simulink model "AutomotiveEMS"  (R2018a)
settings: Solver=VariableStepAuto  StartTime=0  StopTime=3.5  FixedStep=1e-6
undefined symbols (not defined in the file): alternator, buck, DiscIntNeverNeededParam, electrical_load, hybrid_control, i_f_max, iceToAltRotRatio, n_ice_f, n_ice_i, rectifier, t_brake_f, t_brake_i, T_k, T_r, T_s
libraries: fl_lib x43, nesl_utility x41, elec_lib x33, simulink x10, SimscapeCustomBlocks_lib x2, dsparch4 x2, pe_lib x1
(part 1 of 3)
settings Model: Creator=gabrielrodrigues  LastModifiedBy=gabriel.rodrigues
settings DataIOCC: ReturnWorkspaceOutputs=on
settings CodeAppCC: StateflowObjectComments=on
settings SimscapeCC: SimscapeNormalizeSystem=off  SimscapeLogType=local  SimscapeLogLimitData=off

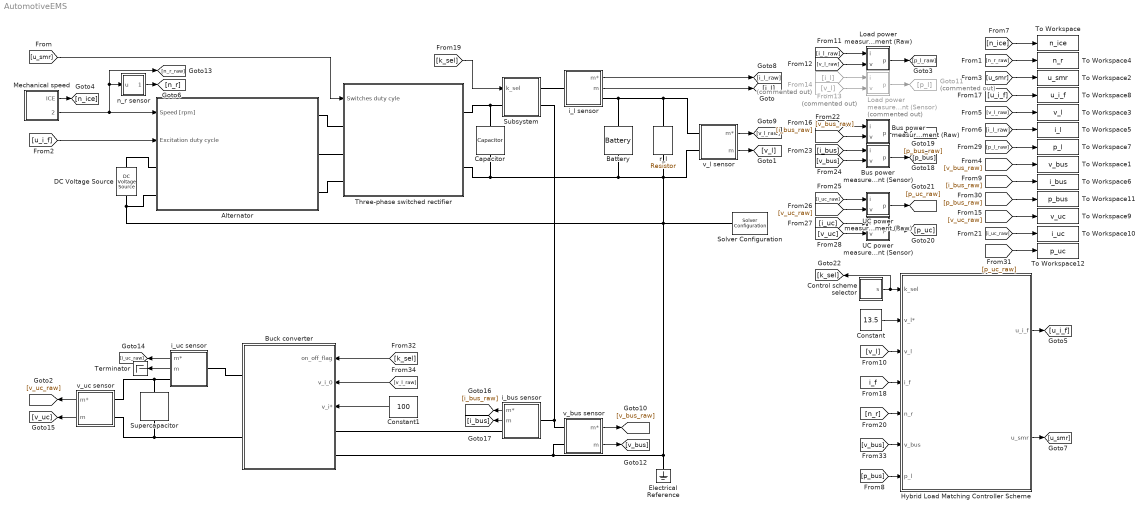
== system AutomotiveEMS ==
  Alternator : Subsystem
  Battery : elec_lib/Sources/Battery  Vnom=battery.v_nom V  R1=battery.r Ohm  prm_AH=2  AH=120 hr*A  V1=11.5 V  AH1=25 hr*A  prm_R2=1  R2=2000 Ohm  prm_dyn=1  Rp1=0.005 Ohm  tau1=30 s  Rp2=0.005 Ohm  tau2=30 s  Rp3=0.005 Ohm  tau3=30 s  Rp4=0.005 Ohm  tau4=30 s  Rp5=0.005 Ohm  tau5=30 s  prm_fade=1  N_fade=100  AH_fade=45 hr*A  R1_fade=2.02 Ohm  V1_fade=10.35 V  i_specify=off  i_priority=None  i=0 A  i_nominal_specify=off  i_nominal_unit=A  i_nominal_value=1  v_specify=off  v_priority=None  v=0 V  v_nominal_specify=off  v_nominal_unit=V  v_nominal_value=1  charge_specify=off  charge_priority=High  charge=50 hr*A  charge_nominal_specify=off  charge_nominal_unit=hr*A  charge_nominal_value=1  num_cycles_specify=off  num_cycles_priority=High  num_cycles=0  num_cycles_nominal_specify=off  num_cycles_nominal_unit=1  num_cycles_nominal_value=1  thermal_mass=30000 J/K  Tmeas=298.15 K  Vnom_T2=12 V  R1_T2=2.2 Ohm  V1_T2=11.4 V  R2_T2=2200 Ohm  Rp1_T2=0.005 Ohm  tau1_T2=30 s  Rp2_T2=0.005 Ohm  tau2_T2=30 s  Rp3_T2=0.005 Ohm  tau3_T2=30 s  Rp4_T2=0.005 Ohm  tau4_T2=30 s  Rp5_T2=0.005 Ohm  tau5_T2=30 s  Tmeas2=273.15 K  temperature_specify=off  temperature_priority=High  temperature=298.15 K  temperature_nominal_specify=off  temperature_nominal_unit=K  temperature_nominal_value=1
      settings: SourceProductName=Simscape Electronics  SourceProductBaseCode=SN
  Buck converter : Subsystem  mask{eta=buck.efficiency, v_o_max=buck.v_o_max}
      mask prompts: eta "Converter efficiency"; v_o_max "Maximum output voltage [V]"
  Bus power measurement (Raw) : Subsystem
  Bus power measurement (Sensor) : Subsystem
  Capacitor : fl_lib/Electrical/Electrical Elements/Capacitor  c=rectifier.filter.c F  r=1e-6 Ohm  g=0 1/Ohm  i_specify=off  i_priority=None  i=0 A  i_nominal_specify=off  i_nominal_unit=A  i_nominal_value=1  v_specify=off  v_priority=None  v=0 V  v_nominal_specify=off  v_nominal_unit=V  v_nominal_value=1  vc_specify=off  vc_priority=High  vc=0 V  vc_nominal_specify=off  vc_nominal_unit=V  vc_nominal_value=1
  Constant : Constant  Value=13.5
  Constant1 : Constant  Value=100
  Control scheme selector : Subsystem  mask{s_i=0, s_f=1, t_i=t_brake_i, t_f=t_brake_f}
      mask prompts: s_i "Initial value"; s_f "Final value"; t_i "Step start [s]"; t_f "Step end [s]"
  DC Voltage Source : elec_lib/Additional Components/SPICE-Compatible Components/Sources/DC Voltage Source  DC=alternator.rotor.r.value * i_f_max V
      settings: SourceProductName=Simscape Electronics  SourceProductBaseCode=SN
  Electrical Reference : fl_lib/Electrical/Electrical Elements/Electrical Reference
  From13 : From  Commented=on  GotoTag=i_l
  From14 : From  Commented=on  GotoTag=v_l
  Goto11 : Goto  Commented=on  GotoTag=p_l
  Hybrid Load Matching Controller Scheme : Subsystem  VariantControl=neural3InControlScheme
  Load power measurement (Raw) : Subsystem
  Load power measurement (Sensor) : Subsystem  Commented=on
  Mechanical speed : Subsystem
  Solver Configuration : nesl_utility/Solver Configuration  PhysicalDomain=network_engine_domain  SubClassName=solver  LeftPortType=input  RightPortType=generic  Tones=[]  Harmonics=[]  SimulateNoise=off  Profile=off  UseLocalSampling=off  EnableSwitchedLinearOptims=on  FrequencyDomain=off  UseCCode=off  RelTol=0.001  AbsTol=1e-06  MinStep=1e-09  ToWorkspace=off  RevertToSquareIcSolve=off  NumHomotopyIterations=100  PhasorMode=off  PhasorModeNumHarmonics=1  DoDC=off  ResidualTolerance=1e-09  UseLocalSolver=on  LocalSolverChoice=NE_TRAPEZOIDAL_ADVANCER  LocalSolverSampleTime=1e-06  DoFixedCost=on  MaxNonlinIter=20  MaxModeIter=2  LinearAlgebra=Sparse  EquationFormulation=NE_TIME_EF  DelaysMemoryBudget=1024  AutomaticFiltering=on  FilteringTimeConstant=0.001  PartitionStorageMethod=AS_NEEDED  PartitionMemoryBudget=1024
  Subsystem : Subsystem
  Supercapacitor : pe_lib/Sources/Supercapacitor  R=[1.5e-3, 0.4, 3.2] Ohm  C=[900, 200, 330] F  Kv=600 F/V  R_discharge=4e+3 Ohm  N_series=6  N_parallel=4  i_specify=off  i_priority=None  i=0 A  i_nominal_specify=off  i_nominal_unit=A  i_nominal_value=1  v_specify=off  v_priority=None  v=0 V  v_nominal_specify=off  v_nominal_unit=V  v_nominal_value=1  vc1_specify=off  vc1_priority=High  vc1=0 V  vc1_nominal_specify=off  vc1_nominal_unit=V  vc1_nominal_value=1  vc2_specify=off  vc2_priority=High  vc2=0 V  vc2_nominal_specify=off  vc2_nominal_unit=V  vc2_nominal_value=1  vc3_specify=off  vc3_priority=High  vc3=0 V  vc3_nominal_specify=off  vc3_nominal_unit=V  vc3_nominal_value=1
      settings: SourceProductName=Simscape Electrical  SourceProductBaseCode=PS
  Terminator : Terminator
  Three-phase switched rectifier : Subsystem
  To Workspace : ToWorkspace  VariableName=n_ice  SaveFormat=Timeseries  SampleTime=-1
  To Workspace1 : ToWorkspace  VariableName=v_bus  SaveFormat=Timeseries  SampleTime=-1
  To Workspace10 : ToWorkspace  VariableName=i_uc  SaveFormat=Timeseries  SampleTime=-1
  To Workspace11 : ToWorkspace  VariableName=p_bus  SaveFormat=Timeseries  SampleTime=-1
  To Workspace12 : ToWorkspace  VariableName=p_uc  SaveFormat=Timeseries  SampleTime=-1
  To Workspace2 : ToWorkspace  VariableName=u_smr  SaveFormat=Timeseries  SampleTime=-1
  To Workspace3 : ToWorkspace  VariableName=v_l  SaveFormat=Timeseries  SampleTime=-1
  To Workspace4 : ToWorkspace  VariableName=n_r  SaveFormat=Timeseries  SampleTime=-1
  To Workspace5 : ToWorkspace  VariableName=i_l  SaveFormat=Timeseries  SampleTime=-1
  To Workspace6 : ToWorkspace  VariableName=i_bus  SaveFormat=Timeseries  SampleTime=-1
  To Workspace7 : ToWorkspace  VariableName=p_l  SaveFormat=Timeseries  SampleTime=-1
  To Workspace8 : ToWorkspace  VariableName=u_i_f  SaveFormat=Timeseries  SampleTime=-1
  To Workspace9 : ToWorkspace  VariableName=v_uc  SaveFormat=Timeseries  SampleTime=-1
  UC power measurement (Raw) : Subsystem
  UC power measurement (Sensor) : Subsystem
  i_bus sensor : Subsystem
  i_l sensor : Subsystem
  i_uc sensor : Subsystem
  n_r sensor : Subsystem  mask{T_s=T_s, seed=1515, noise=0.001}
      mask prompts: T_s "Sample time [s]"; noise "Noise percentage"
      mask DialogControl DescGroupVar Prompt: Noisy voltage sensor
  r_l : elec_lib/Passive Devices/Resistor  R=electrical_load.r Ohm  R_tol=5  enable_R_tol=0  tol_distribution=1  nSigma=4  enable_operating_limits=0  operating_limit_action=2  max_working_voltage=100 V  power_rating=1 W  enable_faults=0  fault_action=1  R_faulted=inf Ohm  enable_temporal_fault=0  t_fault=1 s  enable_behavioral_fault=0  max_permissible_current=1 A  t_fail_on_current=1 s  noise_mode=0  sample_time=1e-3 s  repeatability=1  auto_seed=2238261350  user_seed=0  Tdevice=25 degC  alpha=3.93e-3 1/K  Tmeas=25 degC  thermal_mass=100 J/K  power_derating_T1=70 degC  power_derating_T2=155 degC  operating_temperature_range_vec=[-50, 150] degC  temperature_specify=off  temperature_priority=High  temperature=298.15 K  temperature_nominal_specify=off  temperature_nominal_unit=K  temperature_nominal_value=1
  v_bus sensor : Subsystem
  v_l sensor : Subsystem
  v_uc sensor : Subsystem
  wires:
  Mechanical speed/2(Alternator) -> Alternator/1(Speed [rpm]), [n_r_raw], n_r sensor/1(u)
  n_r sensor/1(m) -> [n_r]
  i_l sensor/2(m) -> [i_l]
  Hybrid Load Matching Controller Scheme/1(u_i_f) -> [u_i_f]
  v_l sensor/1(m*) -> [v_l_raw]
  [u_smr] -> Three-phase switched rectifier/1(Switches duty cyle)
  v_l sensor/2(m) -> [v_l]
  Hybrid Load Matching Controller Scheme/2(u_smr) -> [u_smr]
  Mechanical speed/1(ICE) -> [n_ice]
  i_l sensor/1(m*) -> [i_l_raw]
  [u_i_f] -> To Workspace8/1
  [u_smr] -> To Workspace2/1
  [v_l_raw] -> To Workspace3/1
  [n_ice] -> To Workspace/1
  [n_r_raw] -> To Workspace4/1
  [i_l_raw] -> To Workspace5/1
  [k_sel] -> Subsystem/1(k_sel)
  [p_bus] -> Hybrid Load Matching Controller Scheme/7(p_l)
  Constant/1 -> Hybrid Load Matching Controller Scheme/2(v_l*)
  [v_l] -> Hybrid Load Matching Controller Scheme/3(v_l)
  [n_r] -> Hybrid Load Matching Controller Scheme/5(n_r)
  Load power measurement (Sensor)/1(p) -> Goto11/1
  From13/1 -> Load power measurement (Sensor)/1(i)
  [v_l_raw] -> Load power measurement (Raw)/2(v)
  Load power measurement (Raw)/1(p) -> [p_l_raw]
  From14/1 -> Load power measurement (Sensor)/2(v)
  [i_l_raw] -> Load power measurement (Raw)/1(i)
  v_uc sensor/1(m*) -> [v_uc_raw]
  v_uc sensor/2(m) -> [v_uc]
  v_bus sensor/1(m*) -> [v_bus_raw]
  v_bus sensor/2(m) -> [v_bus]
  i_uc sensor/1(m*) -> [i_uc_raw]
  i_uc sensor/2(m) -> Terminator/1
  [i_bus_raw] -> To Workspace6/1
  [v_bus_raw] -> To Workspace1/1
  [i_uc_raw] -> To Workspace10/1
  [v_uc_raw] -> To Workspace9/1
  i_bus sensor/1(m*) -> [i_bus_raw]
  i_bus sensor/2(m) -> [i_bus]
  [i_bus_raw] -> Bus power measurement (Raw)/1(i)
  Bus power measurement (Raw)/1(p) -> [p_bus_raw]
  [v_bus] -> Bus power measurement (Sensor)/2(v)
  [v_bus_raw] -> Bus power measurement (Raw)/2(v)
  [i_bus] -> Bus power measurement (Sensor)/1(i)
  Bus power measurement (Sensor)/1(p) -> [p_bus]
  [i_uc_raw] -> UC power measurement (Raw)/1(i)
  UC power measurement (Raw)/1(p) -> [p_uc_raw]
  [v_uc] -> UC power measurement (Sensor)/2(v)
  [v_uc_raw] -> UC power measurement (Raw)/2(v)
  [i_uc] -> UC power measurement (Sensor)/1(i)
  UC power measurement (Sensor)/1(p) -> [p_uc]
  [p_l_raw] -> To Workspace7/1
  [p_bus_raw] -> To Workspace11/1
  [p_uc_raw] -> To Workspace12/1
  Control scheme selector/1(s) -> [k_sel], Hybrid Load Matching Controller Scheme/1(k_sel)
  [k_sel] -> Buck converter/1(on_off_flag)
  [u_i_f] -> Alternator/2(Excitation duty cycle)
  [i_f] -> Hybrid Load Matching Controller Scheme/4(i_f)
  [v_bus] -> Hybrid Load Matching Controller Scheme/6(v_bus)
  [v_l_raw] -> Buck converter/2(v_i_0)
  Constant1/1 -> Buck converter/3(v_i*)
  connections:
  Three-phase switched rectifier/RConn2 -- Capacitor/RConn1 -- Battery/RConn1 -- v_l sensor/LConn2 -- v_bus sensor/LConn2 -- Buck converter/LConn2 -- Electrical Reference/LConn1 -- Solver Configuration/RConn1 -- DC Voltage Source/RConn1 -- Alternator/LConn2 -- r_l/RConn1
  Battery/LConn1 -- i_l sensor/RConn1 -- v_l sensor/LConn1 -- r_l/LConn1
  DC Voltage Source/LConn1 -- Alternator/LConn1
  Three-phase switched rectifier/LConn1 -- Alternator/RConn1
  Three-phase switched rectifier/LConn2 -- Alternator/RConn2
  Three-phase switched rectifier/LConn3 -- Alternator/RConn3
  i_l sensor/LConn1 -- Subsystem/RConn1
  Subsystem/LConn1 -- Capacitor/LConn1 -- Three-phase switched rectifier/RConn1
  i_uc sensor/RConn1 -- Supercapacitor/LConn1 -- v_uc sensor/LConn1
  v_uc sensor/LConn2 -- Supercapacitor/RConn1 -- Buck converter/RConn2
  Buck converter/RConn1 -- i_uc sensor/LConn1
  i_bus sensor/LConn1 -- Subsystem/RConn2 -- v_bus sensor/LConn1
  Buck converter/LConn1 -- i_bus sensor/RConn1

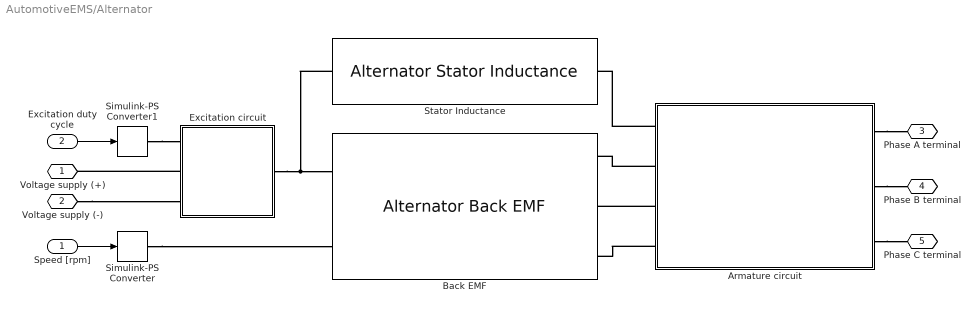
== system AutomotiveEMS/Alternator ==
  Speed [rpm] : Inport
  Excitation duty cycle : Inport  Port=2
  Armature circuit : Subsystem  Variant=on
  Back EMF : SimscapeCustomBlocks_lib/Alternator/Alternator Back EMF  p=alternator.p  omega_r_specify=off  omega_r_priority=None  omega_r=0 rad/s  omega_r_nominal_specify=off  omega_r_nominal_unit=rad/s  omega_r_nominal_value=1  omega_e_specify=off  omega_e_priority=None  omega_e=0 rad/s  omega_e_nominal_specify=off  omega_e_nominal_unit=rad/s  omega_e_nominal_value=1  theta_e_specify=off  theta_e_priority=None  theta_e=0 rad  theta_e_nominal_specify=off  theta_e_nominal_unit=rad  theta_e_nominal_value=1  k_e_specify=off  k_e_priority=None  k_e=0 s*V/rad/A  k_e_nominal_specify=off  k_e_nominal_unit=s*V/rad/A  k_e_nominal_value=1  e_specify=off  e_priority=None  e=0 rpm  e_nominal_specify=off  e_nominal_unit=rpm  e_nominal_value=1
  Excitation circuit : Subsystem
  Simulink-PS Converter : nesl_utility/Simulink-PS Converter  PhysicalDomain=network_engine_domain  SubClassName=ps_input  LeftPortType=input  RightPortType=output  PseudoPeriodic=off  Frequencies=[]  NoiseDistribution=none  NoiseParameters=[]  Unit=1  AffineConversion=off  FilteringAndDerivatives=provide  SimscapeFilterOrder=1  InputFilterTimeConstant=0.001  UdotUserProvided=0
  Simulink-PS Converter1 : nesl_utility/Simulink-PS Converter  PhysicalDomain=network_engine_domain  SubClassName=ps_input  LeftPortType=input  RightPortType=output  PseudoPeriodic=off  Frequencies=[]  NoiseDistribution=none  NoiseParameters=[]  Unit=1  AffineConversion=off  FilteringAndDerivatives=provide  SimscapeFilterOrder=1  InputFilterTimeConstant=0.001  UdotUserProvided=0
  Stator Inductance : SimscapeCustomBlocks_lib/Alternator/Alternator Stator Inductance
  Voltage supply (+) : PMIOPort  Side=Left
  Voltage supply (-) : PMIOPort  Port=2  Side=Left
  Phase A terminal : PMIOPort  Port=3  Side=Right
  Phase B terminal : PMIOPort  Port=4  Side=Right
  Phase C terminal : PMIOPort  Port=5  Side=Right
  wires:
  Speed [rpm]/1 -> Simulink-PS Converter/1
  Excitation duty cycle/1 -> Simulink-PS Converter1/1
  connections:
  Armature circuit/RConn1 -- Phase A terminal/RConn1
  Armature circuit/RConn2 -- Phase B terminal/RConn1
  Excitation circuit/LConn2 -- Voltage supply (+)/RConn1
  Voltage supply (-)/RConn1 -- Excitation circuit/LConn3
  Armature circuit/LConn3 -- Back EMF/RConn2
  Armature circuit/LConn2 -- Back EMF/RConn1
  Armature circuit/LConn4 -- Back EMF/RConn3
  Simulink-PS Converter/RConn1 -- Back EMF/LConn2
  Armature circuit/LConn1 -- Stator Inductance/RConn1
  Excitation circuit/RConn1 -- Stator Inductance/LConn1 -- Back EMF/LConn1
  Armature circuit/RConn3 -- Phase C terminal/RConn1
  Simulink-PS Converter1/RConn1 -- Excitation circuit/LConn1

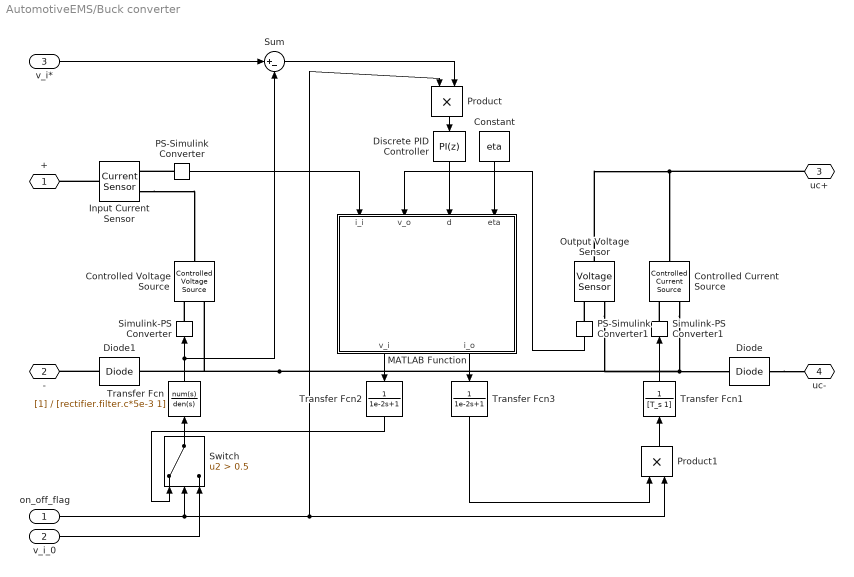
== system AutomotiveEMS/Buck converter ==
  on_off_flag : Inport
  v_i_0 : Inport  Port=2
  v_i* : Inport  Port=3
  Constant : Constant  Value=eta
  Controlled Current Source : fl_lib/Electrical/Electrical Sources/Controlled Current Source
  Controlled Voltage Source : fl_lib/Electrical/Electrical Sources/Controlled Voltage Source
  Diode : elec_lib/Semiconductor Devices/Diode  ModelType=1  Vf=1e-9 V  Ron=1e-9 Ohm  Goff=1e-8 S  Rz=0.3 Ohm  Vz=50 V  C_PWL=5 pF  prmExp=1  I12=[.0137, .545] A  V12=[.6, .7] V  I1=0.0137 A  V1=0.6 V  IS=1e-12 A  ec=1  RS=0.01 Ohm  Tmeas=25 degC  BV=inf V  C_param=1  CJ0=5 pF  VJ=1 V  Mgrad=0.5  Vvec=[.1, 10, 100] V  Cvec=[3.5, 1, .4] pF  FC=0.5  Q_param=1  Irrm=-7.15 A  iF=4 A  didt=-750 A/us  trr=115 ns  TT=50 ns  tau=100 ns  T_param=1  IS_T2=1.25e-7 A  I1_T2=0.245 A  V1_T2=0.5 V  Tmeas2=125 degC  EG_param=1  EG=1.11 eV  XTI_param=1  XTI=3  dBVdT=0 V/K  Tdevice=25 degC  i_capacitor_specify=off  i_capacitor_priority=High  i_capacitor=0 A  i_capacitor_nominal_specify=off  i_capacitor_nominal_unit=A  i_capacitor_nominal_value=1  v_capacitor_specify=off  v_capacitor_priority=None  v_capacitor=0 V  v_capacitor_nominal_specify=off  v_capacitor_nominal_unit=V  v_capacitor_nominal_value=1  Rth=[0, 10] K/W  thermal_mass_parameterization=1  thermal_mass=[0, 1] J/K  thermal_time_constant=[0, 10] s  thermal_mass_initial_temperatures=[25, 25] degC
      settings: SourceProductName=Simscape Electronics  SourceProductBaseCode=SN
  Diode1 : elec_lib/Semiconductor Devices/Diode  ModelType=1  Vf=1e-9 V  Ron=1e-9 Ohm  Goff=1e-8 S  Rz=0.3 Ohm  Vz=50 V  C_PWL=5 pF  prmExp=1  I12=[.0137, .545] A  V12=[.6, .7] V  I1=0.0137 A  V1=0.6 V  IS=1e-12 A  ec=1  RS=0.01 Ohm  Tmeas=25 degC  BV=inf V  C_param=1  CJ0=5 pF  VJ=1 V  Mgrad=0.5  Vvec=[.1, 10, 100] V  Cvec=[3.5, 1, .4] pF  FC=0.5  Q_param=1  Irrm=-7.15 A  iF=4 A  didt=-750 A/us  trr=115 ns  TT=50 ns  tau=100 ns  T_param=1  IS_T2=1.25e-7 A  I1_T2=0.245 A  V1_T2=0.5 V  Tmeas2=125 degC  EG_param=1  EG=1.11 eV  XTI_param=1  XTI=3  dBVdT=0 V/K  Tdevice=25 degC  i_capacitor_specify=off  i_capacitor_priority=High  i_capacitor=0 A  i_capacitor_nominal_specify=off  i_capacitor_nominal_unit=A  i_capacitor_nominal_value=1  v_capacitor_specify=off  v_capacitor_priority=None  v_capacitor=0 V  v_capacitor_nominal_specify=off  v_capacitor_nominal_unit=V  v_capacitor_nominal_value=1  Rth=[0, 10] K/W  thermal_mass_parameterization=1  thermal_mass=[0, 1] J/K  thermal_time_constant=[0, 10] s  thermal_mass_initial_temperatures=[25, 25] degC
      settings: SourceProductName=Simscape Electronics  SourceProductBaseCode=SN
  Discrete PID Controller : simulink/Continuous/PID Controller  Controller=PI  Form=Parallel  TimeDomain=Discrete-time  SampleTime=T_k  IntegratorMethod=Trapezoidal  FilterMethod=Forward Euler  ControllerParametersSource=internal  P=-0.01  I=-0.005  D=0  UseFilter=on  N=100  TunerSelectOption=Transfer Function Based (PID Tuner App)  InitialConditionSource=internal  InitialConditionForIntegrator=0  InitialConditionForFilter=0  DifferentiatorICPrevScaledInput=0  ExternalReset=none  TrackingMode=off  Kt=1  LimitOutput=on  UpperSaturationLimit=0.70  LowerSaturationLimit=0.1/13.5  LinearizeAsGain=off  AntiWindupMode=clamping  Kb=1  POutMin=[]  POutMax=[]  IOutMin=[]  IOutMax=[]  DOutMin=[]  DOutMax=[]  NOutMin=[]  NOutMax=[]  SumOutMin=[]  SumOutMax=[]  SaturationOutMin=[]  SaturationOutMax=[]  PParamMin=[]  PParamMax=[]  IParamMin=[]  IParamMax=[]  DParamMin=[]  DParamMax=[]  NParamMin=[]  NParamMax=[]  KbParamMin=[]  KbParamMax=[]  KtParamMin=[]  KtParamMax=[]  KbOutMin=[]  KbOutMax=[]  KtOutMin=[]  KtOutMax=[]  IntegratorOutMin=[]  IntegratorOutMax=[]  FilterOutMin=[]  FilterOutMax=[]  SumI1OutMin=[]  SumI1OutMax=[]  SumI2OutMin=[]  SumI2OutMax=[]  SumI3OutMin=[]  SumI3OutMax=[]  SumDOutMin=[]  SumDOutMax=[]  DifferentiatorOutMin=[]  DifferentiatorOutMax=[]  FilterDiffOutCoefMin=[]  FilterDiffOutCoefMax=[]  ReciprocalOutMin=[]  ReciprocalOutMax=[]  SumDenOutMin=[]  SumDenOutMax=[]  SumNumOutMin=[]  SumNumOutMax=[]  DivideOutMin=[]  DivideOutMax=[]  IntegratorContinuousStateAttributes=''  IntegratorStateMustResolveToSignalObject=off  IntegratorRTWStateStorageClass=Auto  FilterContinuousStateAttributes=''  FilterStateMustResolveToSignalObject=off  FilterRTWStateStorageClass=Auto
  Input Current Sensor : fl_lib/Electrical/Electrical Sensors/Current Sensor
  MATLAB Function : MATLAB Function  TreatAsAtomicUnit=on
  Output Voltage Sensor : fl_lib/Electrical/Electrical Sensors/Voltage Sensor
  PS-Simulink Converter : nesl_utility/PS-Simulink Converter  PhysicalDomain=network_engine_domain  SubClassName=ps_output  LeftPortType=input  RightPortType=output  PseudoPeriodic=off  Frequencies=[]  Unit=1  AffineConversion=off
  PS-Simulink Converter1 : nesl_utility/PS-Simulink Converter  PhysicalDomain=network_engine_domain  SubClassName=ps_output  LeftPortType=input  RightPortType=output  PseudoPeriodic=off  Frequencies=[]  Unit=1  AffineConversion=off
  Product : Product
  Product1 : Product
  Simulink-PS Converter : nesl_utility/Simulink-PS Converter  PhysicalDomain=network_engine_domain  SubClassName=ps_input  LeftPortType=input  RightPortType=output  PseudoPeriodic=off  Frequencies=[]  NoiseDistribution=none  NoiseParameters=[]  Unit=1  AffineConversion=off  FilteringAndDerivatives=provide  SimscapeFilterOrder=1  InputFilterTimeConstant=0.001  UdotUserProvided=0
  Simulink-PS Converter1 : nesl_utility/Simulink-PS Converter  PhysicalDomain=network_engine_domain  SubClassName=ps_input  LeftPortType=input  RightPortType=output  PseudoPeriodic=off  Frequencies=[]  NoiseDistribution=none  NoiseParameters=[]  Unit=1  AffineConversion=off  FilteringAndDerivatives=provide  SimscapeFilterOrder=1  InputFilterTimeConstant=0.001  UdotUserProvided=0
  Sum : Sum  Inputs=|+-
  Switch : Switch  Criteria=u2 > Threshold  Threshold=0.5
  Transfer Fcn : TransferFcn  Denominator=[rectifier.filter.c*5e-3 1]
  Transfer Fcn1 : TransferFcn  Denominator=[T_s 1]
  Transfer Fcn2 : TransferFcn  Denominator=[1e-2 1]
  Transfer Fcn3 : TransferFcn  Denominator=[1e-2 1]
  + : PMIOPort  Side=Left
  - : PMIOPort  Port=2  Side=Left
  uc+ : PMIOPort  Port=3  Side=Right
  uc- : PMIOPort  Port=4  Side=Right
  wires:
  Transfer Fcn/1 -> Simulink-PS Converter/1, Sum/2
  Transfer Fcn1/1 -> Simulink-PS Converter1/1
  Constant/1 -> MATLAB Function/4(eta)
  PS-Simulink Converter/1 -> MATLAB Function/1(i_i)
  PS-Simulink Converter1/1 -> MATLAB Function/2(v_o)
  Switch/1 -> Transfer Fcn/1
  on_off_flag/1 -> Product/1, Product1/2, Switch/2
  v_i_0/1 -> Switch/3
  Product1/1 -> Transfer Fcn1/1
  v_i*/1 -> Sum/1
  Product/1 -> Discrete PID Controller/1
  Sum/1 -> Product/2
  MATLAB Function/2(i_o) -> Transfer Fcn3/1
  Discrete PID Controller/1 -> MATLAB Function/3(d)
  MATLAB Function/1(v_i) -> Transfer Fcn2/1
  Transfer Fcn3/1 -> Product1/1
  Transfer Fcn2/1 -> Switch/1
  connections:
  Input Current Sensor/LConn1 -- +/RConn1
  Output Voltage Sensor/LConn1 -- uc+/RConn1 -- Controlled Current Source/LConn1
  Input Current Sensor/RConn2 -- Controlled Voltage Source/LConn1
  Controlled Current Source/RConn2 -- Output Voltage Sensor/RConn2 -- Diode1/LConn1 -- Controlled Voltage Source/RConn2 -- Diode/RConn1
  Simulink-PS Converter/RConn1 -- Controlled Voltage Source/RConn1
  Simulink-PS Converter1/RConn1 -- Controlled Current Source/RConn1
  PS-Simulink Converter/LConn1 -- Input Current Sensor/RConn1
  PS-Simulink Converter1/LConn1 -- Output Voltage Sensor/RConn1
  Diode/LConn1 -- uc-/RConn1
  Diode1/RConn1 -- -/RConn1

== system AutomotiveEMS/Bus power measurement (Raw) ==
  i : Inport
  v : Inport  Port=2
  Product : Product
  p : Outport
  wires:
  Product/1 -> p/1
  i/1 -> Product/1
  v/1 -> Product/2

== system AutomotiveEMS/Bus power measurement (Sensor) ==
  i : Inport
  v : Inport  Port=2
  Product : Product
  p : Outport
  wires:
  Product/1 -> p/1
  i/1 -> Product/1
  v/1 -> Product/2

== system AutomotiveEMS/Control scheme selector ==
  Step off : Step  Time=t_f  After=s_f - s_i  SampleTime=0
  Step on : Step  Time=t_i  Before=s_i  After=s_f  SampleTime=0
  Sum : Sum  Inputs=+-
  s : Outport
  wires:
  Sum/1 -> s/1
  Step off/1 -> Sum/2
  Step on/1 -> Sum/1

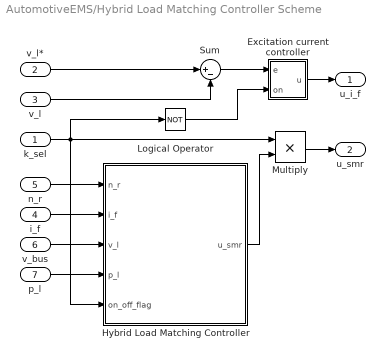
== system AutomotiveEMS/Hybrid Load Matching Controller Scheme ==
  k_sel : Inport
  v_l* : Inport  Port=2
  v_l : Inport  Port=3
  i_f : Inport  Port=4
  n_r : Inport  Port=5
  v_bus : Inport  Port=6
  p_l : Inport  Port=7
  Excitation current controller : Subsystem
  Hybrid Load Matching Controller : Subsystem
  Logical Operator : Logic  Operator=NOT  AllPortsSameDT=off  OutDataTypeStr=boolean
  Multiply : Product
  Sum : Sum  Inputs=|+-
  u_i_f : Outport
  u_smr : Outport  Port=2
  wires:
  Logical Operator/1 -> Excitation current controller/2(on)
  v_bus/1 -> Hybrid Load Matching Controller/3(v_l)
  k_sel/1 -> Hybrid Load Matching Controller/5(on_off_flag), Logical Operator/1, Multiply/1
  Sum/1 -> Excitation current controller/1(e)
  v_l/1 -> Sum/2
  Hybrid Load Matching Controller/1(u_smr) -> Multiply/2
  v_l*/1 -> Sum/1
  Excitation current controller/1(u) -> u_i_f/1
  i_f/1 -> Hybrid Load Matching Controller/2(i_f)
  p_l/1 -> Hybrid Load Matching Controller/4(p_l)
  n_r/1 -> Hybrid Load Matching Controller/1(n_r)
  Multiply/1 -> u_smr/1

== system AutomotiveEMS/Load power measurement (Raw) ==
  i : Inport
  v : Inport  Port=2
  Product : Product
  p : Outport
  wires:
  Product/1 -> p/1
  i/1 -> Product/1
  v/1 -> Product/2

== system AutomotiveEMS/Load power measurement (Sensor) ==
  i : Inport
  v : Inport  Port=2
  Product : Product
  p : Outport
  wires:
  Product/1 -> p/1
  i/1 -> Product/1
  v/1 -> Product/2

== system AutomotiveEMS/Mechanical speed ==
  ICE Speed : Subsystem  mask{s_i=n_ice_i, s_f=n_ice_f, t_i=t_brake_i, t_f=t_brake_f}
      mask prompts: s_i "Initial value"; s_f "Final value"; t_i "Ramp start [s]"; t_f "Ramp end [s]"
  ICE to Alternator Rotation Ratio : Constant  Value=iceToAltRotRatio
  Product : Product
  ICE : Outport
  Alternator : Outport  Port=2
  wires:
  ICE Speed/1(s) -> ICE/1, Product/1
  ICE to Alternator Rotation Ratio/1 -> Product/2
  Product/1 -> Alternator/1

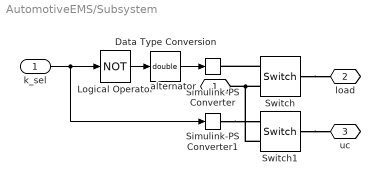
== system AutomotiveEMS/Subsystem ==
  k_sel : Inport
  Data Type Conversion : DataTypeConversion  OutDataTypeStr=double
  Logical Operator : Logic  Operator=NOT  AllPortsSameDT=off  OutDataTypeStr=boolean
  Simulink-PS Converter : nesl_utility/Simulink-PS Converter  PhysicalDomain=network_engine_domain  SubClassName=ps_input  LeftPortType=input  RightPortType=output  PseudoPeriodic=off  Frequencies=[]  NoiseDistribution=none  NoiseParameters=[]  Unit=1  AffineConversion=off  FilteringAndDerivatives=provide  SimscapeFilterOrder=1  InputFilterTimeConstant=0.001  UdotUserProvided=0
  Simulink-PS Converter1 : nesl_utility/Simulink-PS Converter  PhysicalDomain=network_engine_domain  SubClassName=ps_input  LeftPortType=input  RightPortType=output  PseudoPeriodic=off  Frequencies=[]  NoiseDistribution=none  NoiseParameters=[]  Unit=1  AffineConversion=off  FilteringAndDerivatives=provide  SimscapeFilterOrder=1  InputFilterTimeConstant=0.001  UdotUserProvided=0
  Switch : fl_lib/Electrical/Electrical Elements/Switch  R_closed=0.01 Ohm  G_open=1e-8 1/Ohm  Threshold=0.5  i_specify=off  i_priority=None  i=0 A  i_nominal_specify=off  i_nominal_unit=A  i_nominal_value=1  v_specify=off  v_priority=None  v=0 V  v_nominal_specify=off  v_nominal_unit=V  v_nominal_value=1
      settings: SourceProductName=Simscape
  Switch1 : fl_lib/Electrical/Electrical Elements/Switch  R_closed=0.01 Ohm  G_open=1e-8 1/Ohm  Threshold=0.5  i_specify=off  i_priority=None  i=0 A  i_nominal_specify=off  i_nominal_unit=A  i_nominal_value=1  v_specify=off  v_priority=None  v=0 V  v_nominal_specify=off  v_nominal_unit=V  v_nominal_value=1
      settings: SourceProductName=Simscape
  alternator : PMIOPort  Side=Left
  load : PMIOPort  Port=2  Side=Right
  uc : PMIOPort  Port=3  Side=Right
  wires:
  k_sel/1 -> Simulink-PS Converter1/1, Logical Operator/1
  Logical Operator/1 -> Data Type Conversion/1
  Data Type Conversion/1 -> Simulink-PS Converter/1
  connections:
  Switch/LConn1 -- load/RConn1
  Switch/RConn2 -- Switch1/RConn2 -- alternator/RConn1
  Switch/RConn1 -- Simulink-PS Converter/RConn1
  Switch1/LConn1 -- uc/RConn1
  Simulink-PS Converter1/RConn1 -- Switch1/RConn1

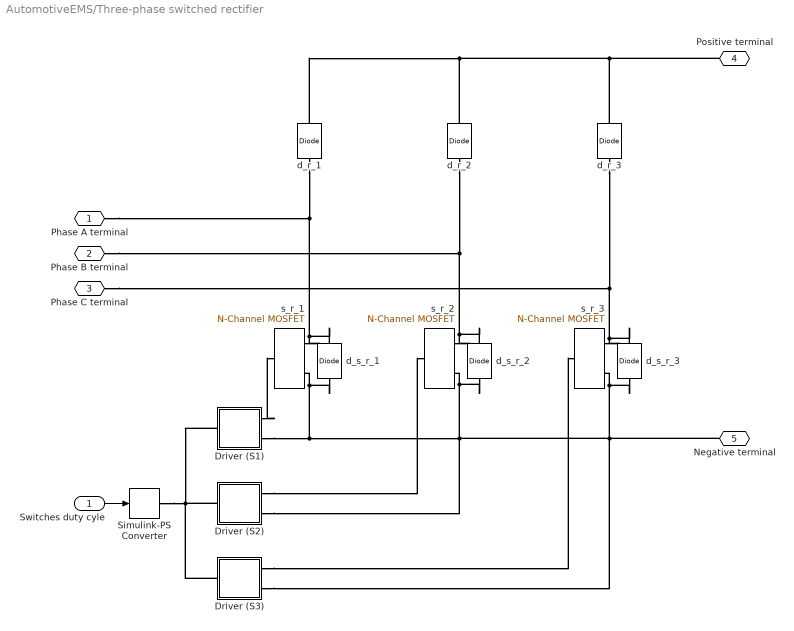
== system AutomotiveEMS/Three-phase switched rectifier ==
  Switches duty cyle : Inport
  Driver (S1) : Subsystem
  Driver (S2) : Subsystem
  Driver (S3) : Subsystem
  Simulink-PS Converter : nesl_utility/Simulink-PS Converter  PhysicalDomain=network_engine_domain  SubClassName=ps_input  LeftPortType=input  RightPortType=output  PseudoPeriodic=off  Frequencies=[]  NoiseDistribution=none  NoiseParameters=[]  Unit=1  AffineConversion=off  FilteringAndDerivatives=provide  SimscapeFilterOrder=1  InputFilterTimeConstant=0.001  UdotUserProvided=0
  d_r_1 : elec_lib/Semiconductor Devices/Diode  ModelType=1  Vf=rectifier.d.v_on V  Ron=rectifier.d.r_on Ohm  Goff=1e-8 S  Rz=0.3 Ohm  Vz=50 V  C_PWL=5 pF  prmExp=1  I12=[.0137, .545] A  V12=[.6, .7] V  I1=0.0137 A  V1=0.6 V  IS=1e-12 A  ec=1  RS=0.01 Ohm  Tmeas=25 degC  BV=inf V  C_param=1  CJ0=5 pF  VJ=1 V  Mgrad=0.5  Vvec=[.1, 10, 100] V  Cvec=[3.5, 1, .4] pF  FC=0.5  Q_param=1  Irrm=-7.15 A  iF=4 A  didt=-750 A/us  trr=115 ns  TT=50 ns  tau=100 ns  T_param=1  IS_T2=1.25e-7 A  I1_T2=0.245 A  V1_T2=0.5 V  Tmeas2=125 degC  EG_param=1  EG=1.11 eV  XTI_param=1  XTI=3  dBVdT=0 V/K  Tdevice=25 degC  i_capacitor_specify=off  i_capacitor_priority=High  i_capacitor=0 A  i_capacitor_nominal_specify=off  i_capacitor_nominal_unit=A  i_capacitor_nominal_value=1  v_capacitor_specify=off  v_capacitor_priority=None  v_capacitor=0 V  v_capacitor_nominal_specify=off  v_capacitor_nominal_unit=V  v_capacitor_nominal_value=1  Rth=[0, 10] K/W  thermal_mass_parameterization=1  thermal_mass=[0, 1] J/K  thermal_time_constant=[0, 10] s  thermal_mass_initial_temperatures=[25, 25] degC
      settings: SourceProductName=Simscape Electronics  SourceProductBaseCode=SN
  d_r_2 : elec_lib/Semiconductor Devices/Diode  ModelType=1  Vf=rectifier.d.v_on V  Ron=rectifier.d.r_on Ohm  Goff=1e-8 S  Rz=0.3 Ohm  Vz=50 V  C_PWL=5 pF  prmExp=1  I12=[.0137, .545] A  V12=[.6, .7] V  I1=0.0137 A  V1=0.6 V  IS=1e-12 A  ec=1  RS=0.01 Ohm  Tmeas=25 degC  BV=inf V  C_param=1  CJ0=5 pF  VJ=1 V  Mgrad=0.5  Vvec=[.1, 10, 100] V  Cvec=[3.5, 1, .4] pF  FC=0.5  Q_param=1  Irrm=-7.15 A  iF=4 A  didt=-750 A/us  trr=115 ns  TT=50 ns  tau=100 ns  T_param=1  IS_T2=1.25e-7 A  I1_T2=0.245 A  V1_T2=0.5 V  Tmeas2=125 degC  EG_param=1  EG=1.11 eV  XTI_param=1  XTI=3  dBVdT=0 V/K  Tdevice=25 degC  i_capacitor_specify=off  i_capacitor_priority=High  i_capacitor=0 A  i_capacitor_nominal_specify=off  i_capacitor_nominal_unit=A  i_capacitor_nominal_value=1  v_capacitor_specify=off  v_capacitor_priority=None  v_capacitor=0 V  v_capacitor_nominal_specify=off  v_capacitor_nominal_unit=V  v_capacitor_nominal_value=1  Rth=[0, 10] K/W  thermal_mass_parameterization=1  thermal_mass=[0, 1] J/K  thermal_time_constant=[0, 10] s  thermal_mass_initial_temperatures=[25, 25] degC
      settings: SourceProductName=Simscape Electronics  SourceProductBaseCode=SN
  d_r_3 : elec_lib/Semiconductor Devices/Diode  ModelType=1  Vf=rectifier.d.v_on V  Ron=rectifier.d.r_on Ohm  Goff=1e-8 S  Rz=0.3 Ohm  Vz=50 V  C_PWL=5 pF  prmExp=1  I12=[.0137, .545] A  V12=[.6, .7] V  I1=0.0137 A  V1=0.6 V  IS=1e-12 A  ec=1  RS=0.01 Ohm  Tmeas=25 degC  BV=inf V  C_param=1  CJ0=5 pF  VJ=1 V  Mgrad=0.5  Vvec=[.1, 10, 100] V  Cvec=[3.5, 1, .4] pF  FC=0.5  Q_param=1  Irrm=-7.15 A  iF=4 A  didt=-750 A/us  trr=115 ns  TT=50 ns  tau=100 ns  T_param=1  IS_T2=1.25e-7 A  I1_T2=0.245 A  V1_T2=0.5 V  Tmeas2=125 degC  EG_param=1  EG=1.11 eV  XTI_param=1  XTI=3  dBVdT=0 V/K  Tdevice=25 degC  i_capacitor_specify=off  i_capacitor_priority=High  i_capacitor=0 A  i_capacitor_nominal_specify=off  i_capacitor_nominal_unit=A  i_capacitor_nominal_value=1  v_capacitor_specify=off  v_capacitor_priority=None  v_capacitor=0 V  v_capacitor_nominal_specify=off  v_capacitor_nominal_unit=V  v_capacitor_nominal_value=1  Rth=[0, 10] K/W  thermal_mass_parameterization=1  thermal_mass=[0, 1] J/K  thermal_time_constant=[0, 10] s  thermal_mass_initial_temperatures=[25, 25] degC
      settings: SourceProductName=Simscape Electronics  SourceProductBaseCode=SN
  d_s_r_1 : elec_lib/Semiconductor Devices/Diode  ModelType=1  Vf=rectifier.d.v_on V  Ron=rectifier.d.r_on Ohm  Goff=1e-8 S  Rz=0.3 Ohm  Vz=50 V  C_PWL=5 pF  prmExp=1  I12=[.0137, .545] A  V12=[.6, .7] V  I1=0.0137 A  V1=0.6 V  IS=1e-12 A  ec=1  RS=0.01 Ohm  Tmeas=25 degC  BV=inf V  C_param=1  CJ0=5 pF  VJ=1 V  Mgrad=0.5  Vvec=[.1, 10, 100] V  Cvec=[3.5, 1, .4] pF  FC=0.5  Q_param=1  Irrm=-7.15 A  iF=4 A  didt=-750 A/us  trr=115 ns  TT=50 ns  tau=100 ns  T_param=1  IS_T2=1.25e-7 A  I1_T2=0.245 A  V1_T2=0.5 V  Tmeas2=125 degC  EG_param=1  EG=1.11 eV  XTI_param=1  XTI=3  dBVdT=0 V/K  Tdevice=25 degC  i_capacitor_specify=off  i_capacitor_priority=High  i_capacitor=0 A  i_capacitor_nominal_specify=off  i_capacitor_nominal_unit=A  i_capacitor_nominal_value=1  v_capacitor_specify=off  v_capacitor_priority=None  v_capacitor=0 V  v_capacitor_nominal_specify=off  v_capacitor_nominal_unit=V  v_capacitor_nominal_value=1  Rth=[0, 10] K/W  thermal_mass_parameterization=1  thermal_mass=[0, 1] J/K  thermal_time_constant=[0, 10] s  thermal_mass_initial_temperatures=[25, 25] degC
      settings: SourceProductName=Simscape Electronics  SourceProductBaseCode=SN
  d_s_r_2 : elec_lib/Semiconductor Devices/Diode  ModelType=1  Vf=rectifier.d.v_on V  Ron=rectifier.d.r_on Ohm  Goff=1e-8 S  Rz=0.3 Ohm  Vz=50 V  C_PWL=5 pF  prmExp=1  I12=[.0137, .545] A  V12=[.6, .7] V  I1=0.0137 A  V1=0.6 V  IS=1e-12 A  ec=1  RS=0.01 Ohm  Tmeas=25 degC  BV=inf V  C_param=1  CJ0=5 pF  VJ=1 V  Mgrad=0.5  Vvec=[.1, 10, 100] V  Cvec=[3.5, 1, .4] pF  FC=0.5  Q_param=1  Irrm=-7.15 A  iF=4 A  didt=-750 A/us  trr=115 ns  TT=50 ns  tau=100 ns  T_param=1  IS_T2=1.25e-7 A  I1_T2=0.245 A  V1_T2=0.5 V  Tmeas2=125 degC  EG_param=1  EG=1.11 eV  XTI_param=1  XTI=3  dBVdT=0 V/K  Tdevice=25 degC  i_capacitor_specify=off  i_capacitor_priority=High  i_capacitor=0 A  i_capacitor_nominal_specify=off  i_capacitor_nominal_unit=A  i_capacitor_nominal_value=1  v_capacitor_specify=off  v_capacitor_priority=None  v_capacitor=0 V  v_capacitor_nominal_specify=off  v_capacitor_nominal_unit=V  v_capacitor_nominal_value=1  Rth=[0, 10] K/W  thermal_mass_parameterization=1  thermal_mass=[0, 1] J/K  thermal_time_constant=[0, 10] s  thermal_mass_initial_temperatures=[25, 25] degC
      settings: SourceProductName=Simscape Electronics  SourceProductBaseCode=SN
  d_s_r_3 : elec_lib/Semiconductor Devices/Diode  ModelType=1  Vf=rectifier.d.v_on V  Ron=rectifier.d.r_on Ohm  Goff=1e-8 S  Rz=0.3 Ohm  Vz=50 V  C_PWL=5 pF  prmExp=1  I12=[.0137, .545] A  V12=[.6, .7] V  I1=0.0137 A  V1=0.6 V  IS=1e-12 A  ec=1  RS=0.01 Ohm  Tmeas=25 degC  BV=inf V  C_param=1  CJ0=5 pF  VJ=1 V  Mgrad=0.5  Vvec=[.1, 10, 100] V  Cvec=[3.5, 1, .4] pF  FC=0.5  Q_param=1  Irrm=-7.15 A  iF=4 A  didt=-750 A/us  trr=115 ns  TT=50 ns  tau=100 ns  T_param=1  IS_T2=1.25e-7 A  I1_T2=0.245 A  V1_T2=0.5 V  Tmeas2=125 degC  EG_param=1  EG=1.11 eV  XTI_param=1  XTI=3  dBVdT=0 V/K  Tdevice=25 degC  i_capacitor_specify=off  i_capacitor_priority=High  i_capacitor=0 A  i_capacitor_nominal_specify=off  i_capacitor_nominal_unit=A  i_capacitor_nominal_value=1  v_capacitor_specify=off  v_capacitor_priority=None  v_capacitor=0 V  v_capacitor_nominal_specify=off  v_capacitor_nominal_unit=V  v_capacitor_nominal_value=1  Rth=[0, 10] K/W  thermal_mass_parameterization=1  thermal_mass=[0, 1] J/K  thermal_time_constant=[0, 10] s  thermal_mass_initial_temperatures=[25, 25] degC
      settings: SourceProductName=Simscape Electronics  SourceProductBaseCode=SN
  s_r_1 : elec_lib/Semiconductor Devices/N-Channel MOSFET  parameterization=1  prmDatasheet=1  prmEquCoeff=1  Beta=5 A/V^2  Rds=0.025 Ohm  Id=6 A  Vgs=rectifier.s.v_gs_on V  Vth=1.7 V  lam=0 1/V  Tmeas=25 degC  RS=1e-4 Ohm  RD=0.01 Ohm  C_param=1  C_GS=270 pF  C_GD=80 pF  C_DS=0 pF  C_iss=350 pF  C_rss=80 pF  C_oss=0 pF  C_GS_vec=[ 270 300 290 280 295 255 ] pF  C_GD_vec=[ 450 400 300 190 95 55 ] pF  C_DS_vec=[ 450 410 390 230 175 115 ] pF  C_iss_vec=[ 720 700 590 470 390 310 ] pF  C_rss_vec=[ 450 400 300 190 95 55 ] pF  C_oss_vec=[ 900 810 690 420 270 170 ] pF  C_Vds_vec=[ 0.1 0.3 1 3 10 30 ] V  V_GS_for_cap_data=0 V  charge_linearity_param=1  C_OX=200 pF  V_C_OX=-0.5 V  IsDiode=0 A  Vbi=0.6 V  n=1  Cj0Diode=0 pF  TT=50e-9 s  dVth_dT=-6 mV/K  Rds_T2=0.037 Ohm  Tmeas2=125 degC  BEXDatasheet=-1.5  BEXEquCoeff=-1.5  etaisDatasheet=3  etaisEquCoeff=3  TdeviceDatasheet=25 degC  TdeviceEquCoeff=25 degC  Rth=[1, 10] K/W  thermal_mass_parameterization=1  thermal_mass=[1, 1] J/K  thermal_time_constant=[1, 10] s  thermal_mass_initial_temperatures=[ 25 25 ] degC  betaref=18 A/V^2  Vfbref=-1.1 V  gamma=3.5 V^0.50000  phib2ref=1 V  thesatref=0.4 1/V  alpha=0  Vp=5e-2 V  thesrref=0 1/V  m=8  Tref=25 degC  Cox=1500 pF  Cgso=100 pF  Cgdo=14 pF  Rsref=2e-3 Ohm  Rdref=0.17 Ohm  Rgref=8.4 Ohm  Isref=5.2e-13 A  Cj0=480 pF  Tprm=1  etabet=1.3  Stvfb=5e-4 V/K  Stphib=-8.5e-4 V/K  etasat=1.04  etasr=0.65  etar=0.95  etais=3  Tsim=25 degC  T0=[25, 25] degC
      settings: SourceProductName=Simscape Electronics  SourceProductBaseCode=SN  LogSimulationData=on
  s_r_2 : elec_lib/Semiconductor Devices/N-Channel MOSFET  parameterization=1  prmDatasheet=1  prmEquCoeff=1  Beta=5 A/V^2  Rds=0.025 Ohm  Id=6 A  Vgs=rectifier.s.v_gs_on V  Vth=1.7 V  lam=0 1/V  Tmeas=25 degC  RS=1e-4 Ohm  RD=0.01 Ohm  C_param=1  C_GS=270 pF  C_GD=80 pF  C_DS=0 pF  C_iss=350 pF  C_rss=80 pF  C_oss=0 pF  C_GS_vec=[ 270 300 290 280 295 255 ] pF  C_GD_vec=[ 450 400 300 190 95 55 ] pF  C_DS_vec=[ 450 410 390 230 175 115 ] pF  C_iss_vec=[ 720 700 590 470 390 310 ] pF  C_rss_vec=[ 450 400 300 190 95 55 ] pF  C_oss_vec=[ 900 810 690 420 270 170 ] pF  C_Vds_vec=[ 0.1 0.3 1 3 10 30 ] V  V_GS_for_cap_data=0 V  charge_linearity_param=1  C_OX=200 pF  V_C_OX=-0.5 V  IsDiode=0 A  Vbi=0.6 V  n=1  Cj0Diode=0 pF  TT=50e-9 s  dVth_dT=-6 mV/K  Rds_T2=0.037 Ohm  Tmeas2=125 degC  BEXDatasheet=-1.5  BEXEquCoeff=-1.5  etaisDatasheet=3  etaisEquCoeff=3  TdeviceDatasheet=25 degC  TdeviceEquCoeff=25 degC  Rth=[1, 10] K/W  thermal_mass_parameterization=1  thermal_mass=[1, 1] J/K  thermal_time_constant=[1, 10] s  thermal_mass_initial_temperatures=[ 25 25 ] degC  betaref=18 A/V^2  Vfbref=-1.1 V  gamma=3.5 V^0.50000  phib2ref=1 V  thesatref=0.4 1/V  alpha=0  Vp=5e-2 V  thesrref=0 1/V  m=8  Tref=25 degC  Cox=1500 pF  Cgso=100 pF  Cgdo=14 pF  Rsref=2e-3 Ohm  Rdref=0.17 Ohm  Rgref=8.4 Ohm  Isref=5.2e-13 A  Cj0=480 pF  Tprm=1  etabet=1.3  Stvfb=5e-4 V/K  Stphib=-8.5e-4 V/K  etasat=1.04  etasr=0.65  etar=0.95  etais=3  Tsim=25 degC  T0=[25, 25] degC
      settings: SourceProductName=Simscape Electronics  SourceProductBaseCode=SN  LogSimulationData=on
  s_r_3 : elec_lib/Semiconductor Devices/N-Channel MOSFET  parameterization=1  prmDatasheet=1  prmEquCoeff=1  Beta=5 A/V^2  Rds=0.025 Ohm  Id=6 A  Vgs=rectifier.s.v_gs_on V  Vth=1.7 V  lam=0 1/V  Tmeas=25 degC  RS=1e-4 Ohm  RD=0.01 Ohm  C_param=1  C_GS=270 pF  C_GD=80 pF  C_DS=0 pF  C_iss=350 pF  C_rss=80 pF  C_oss=0 pF  C_GS_vec=[ 270 300 290 280 295 255 ] pF  C_GD_vec=[ 450 400 300 190 95 55 ] pF  C_DS_vec=[ 450 410 390 230 175 115 ] pF  C_iss_vec=[ 720 700 590 470 390 310 ] pF  C_rss_vec=[ 450 400 300 190 95 55 ] pF  C_oss_vec=[ 900 810 690 420 270 170 ] pF  C_Vds_vec=[ 0.1 0.3 1 3 10 30 ] V  V_GS_for_cap_data=0 V  charge_linearity_param=1  C_OX=200 pF  V_C_OX=-0.5 V  IsDiode=0 A  Vbi=0.6 V  n=1  Cj0Diode=0 pF  TT=50e-9 s  dVth_dT=-6 mV/K  Rds_T2=0.037 Ohm  Tmeas2=125 degC  BEXDatasheet=-1.5  BEXEquCoeff=-1.5  etaisDatasheet=3  etaisEquCoeff=3  TdeviceDatasheet=25 degC  TdeviceEquCoeff=25 degC  Rth=[1, 10] K/W  thermal_mass_parameterization=1  thermal_mass=[1, 1] J/K  thermal_time_constant=[1, 10] s  thermal_mass_initial_temperatures=[ 25 25 ] degC  betaref=18 A/V^2  Vfbref=-1.1 V  gamma=3.5 V^0.50000  phib2ref=1 V  thesatref=0.4 1/V  alpha=0  Vp=5e-2 V  thesrref=0 1/V  m=8  Tref=25 degC  Cox=1500 pF  Cgso=100 pF  Cgdo=14 pF  Rsref=2e-3 Ohm  Rdref=0.17 Ohm  Rgref=8.4 Ohm  Isref=5.2e-13 A  Cj0=480 pF  Tprm=1  etabet=1.3  Stvfb=5e-4 V/K  Stphib=-8.5e-4 V/K  etasat=1.04  etasr=0.65  etar=0.95  etais=3  Tsim=25 degC  T0=[25, 25] degC
      settings: SourceProductName=Simscape Electronics  SourceProductBaseCode=SN  LogSimulationData=on
  Phase A terminal : PMIOPort  Side=Left
  Phase B terminal : PMIOPort  Port=2  Side=Left
  Phase C terminal : PMIOPort  Port=3  Side=Left
  Positive terminal : PMIOPort  Port=4  Side=Right
  Negative terminal : PMIOPort  Port=5  Side=Right
  wires:
  Switches duty cyle/1 -> Simulink-PS Converter/1
  connections:
  Phase B terminal/RConn1 -- d_r_2/LConn1 -- d_s_r_2/RConn1 -- s_r_2/RConn1
  Positive terminal/RConn1 -- d_r_3/RConn1 -- d_r_2/RConn1 -- d_r_1/RConn1
  Phase C terminal/RConn1 -- d_r_3/LConn1 -- d_s_r_3/RConn1 -- s_r_3/RConn1
  Driver (S1)/RConn1 -- s_r_1/LConn1
  Driver (S2)/RConn1 -- s_r_2/LConn1
  Driver (S3)/RConn1 -- s_r_3/LConn1
  Negative terminal/RConn1 -- Driver (S3)/RConn2 -- d_s_r_3/LConn1 -- s_r_3/RConn2 -- Driver (S2)/RConn2 -- Driver (S1)/RConn2 -- d_s_r_1/LConn1 -- s_r_1/RConn2 -- d_s_r_2/LConn1 -- s_r_2/RConn2
  Driver (S3)/LConn1 -- Simulink-PS Converter/RConn1 -- Driver (S2)/LConn1 -- Driver (S1)/LConn1
  d_s_r_1/RConn1 -- Phase A terminal/RConn1 -- d_r_1/LConn1 -- s_r_1/RConn1

== system AutomotiveEMS/UC power measurement (Raw) ==
  i : Inport
  v : Inport  Port=2
  Product : Product
  p : Outport
  wires:
  Product/1 -> p/1
  i/1 -> Product/1
  v/1 -> Product/2

== system AutomotiveEMS/UC power measurement (Sensor) ==
  i : Inport
  v : Inport  Port=2
  Product : Product
  p : Outport
  wires:
  Product/1 -> p/1
  i/1 -> Product/1
  v/1 -> Product/2

== system AutomotiveEMS/i_bus sensor ==
  Current Sensor : Subsystem  mask{T_s=T_r, seed=0, noise=0.01}
      mask prompts: T_s "Sample time [s]"; noise "Noise percentage"
      mask DialogControl DescGroupVar Prompt: Noisy current sensor
  Sample delay1 : TransferFcn  Denominator=[T_s 1]
  Sample delay2 : TransferFcn  Denominator=[T_s 1]
  + : PMIOPort  Side=Left
  - : PMIOPort  Port=2  Side=Right
  m* : Outport
  m : Outport  Port=2
  wires:
  Current Sensor/1(m*) -> Sample delay2/1
  Current Sensor/2(m) -> Sample delay1/1
  Sample delay1/1 -> m/1
  Sample delay2/1 -> m*/1
  connections:
  Current Sensor/RConn1 -- -/RConn1
  Current Sensor/LConn1 -- +/RConn1

== system AutomotiveEMS/i_l sensor ==
  Current Sensor : Subsystem  mask{T_s=T_r, seed=0, noise=0.01}
      mask prompts: T_s "Sample time [s]"; noise "Noise percentage"
      mask DialogControl DescGroupVar Prompt: Noisy current sensor
  Sample delay1 : TransferFcn  Denominator=[T_s 1]
  Sample delay2 : TransferFcn  Denominator=[T_s 1]
  + : PMIOPort  Side=Left
  - : PMIOPort  Port=2  Side=Right
  m* : Outport
  m : Outport  Port=2
  wires:
  Current Sensor/1(m*) -> Sample delay2/1
  Current Sensor/2(m) -> Sample delay1/1
  Sample delay1/1 -> m/1
  Sample delay2/1 -> m*/1
  connections:
  Current Sensor/RConn1 -- -/RConn1
  Current Sensor/LConn1 -- +/RConn1

== system AutomotiveEMS/i_uc sensor ==
  Current Sensor : Subsystem  mask{T_s=T_r, seed=0, noise=0.01}
      mask prompts: T_s "Sample time [s]"; noise "Noise percentage"
      mask DialogControl DescGroupVar Prompt: Noisy current sensor
  Sample delay1 : TransferFcn  Denominator=[T_s 1]
  Sample delay2 : TransferFcn  Denominator=[T_s 1]
  + : PMIOPort  Side=Left
  - : PMIOPort  Port=2  Side=Right
  m* : Outport
  m : Outport  Port=2
  wires:
  Current Sensor/1(m*) -> Sample delay2/1
  Current Sensor/2(m) -> Sample delay1/1
  Sample delay1/1 -> m/1
  Sample delay2/1 -> m*/1
  connections:
  Current Sensor/RConn1 -- -/RConn1
  Current Sensor/LConn1 -- +/RConn1

== system AutomotiveEMS/n_r sensor ==
  u : Inport
  Noise addition : Subsystem  mask{T_s=T_s, seed=seed, noise=noise}
      mask prompts: T_s "Sample time [s]"; noise "Noise percentage"
  m : Outport
  wires:
  Noise addition/1(u + n) -> m/1
  u/1 -> Noise addition/1(u)

== system AutomotiveEMS/v_bus sensor ==
  Sample delay : TransferFcn  Denominator=[T_s 1]
  Sample delay1 : TransferFcn  Denominator=[T_s 1]
  Voltage Sensor : Subsystem  mask{T_s=T_r, seed=15151, noise=0.01}
      mask prompts: T_s "Sample time [s]"; noise "Noise percentage"
      mask DialogControl DescGroupVar Prompt: Noisy voltage sensor
  + : PMIOPort  Side=Left
  - : PMIOPort  Port=2  Side=Left
  m* : Outport
  m : Outport  Port=2
  wires:
  Sample delay/1 -> m*/1
  Sample delay1/1 -> m/1
  Voltage Sensor/2(m) -> Sample delay1/1
  Voltage Sensor/1(m*) -> Sample delay/1
  connections:
  -/RConn1 -- Voltage Sensor/LConn2
  +/RConn1 -- Voltage Sensor/LConn1

== system AutomotiveEMS/v_l sensor ==
  Sample delay : TransferFcn  Denominator=[T_s 1]
  Sample delay1 : TransferFcn  Denominator=[T_s 1]
  Voltage Sensor : Subsystem  mask{T_s=T_r, seed=15151, noise=0.01}
      mask prompts: T_s "Sample time [s]"; noise "Noise percentage"
      mask DialogControl DescGroupVar Prompt: Noisy voltage sensor
  + : PMIOPort  Side=Left
  - : PMIOPort  Port=2  Side=Left
  m* : Outport
  m : Outport  Port=2
  wires:
  Sample delay/1 -> m*/1
  Sample delay1/1 -> m/1
  Voltage Sensor/2(m) -> Sample delay1/1
  Voltage Sensor/1(m*) -> Sample delay/1
  connections:
  -/RConn1 -- Voltage Sensor/LConn2
  +/RConn1 -- Voltage Sensor/LConn1

== system AutomotiveEMS/v_uc sensor ==
  Sample delay : TransferFcn  Denominator=[T_s 1]
  Sample delay1 : TransferFcn  Denominator=[T_s 1]
  Voltage Sensor : Subsystem  mask{T_s=T_r, seed=15151, noise=0.01}
      mask prompts: T_s "Sample time [s]"; noise "Noise percentage"
      mask DialogControl DescGroupVar Prompt: Noisy voltage sensor
  + : PMIOPort  Side=Left
  - : PMIOPort  Port=2  Side=Left
  m* : Outport
  m : Outport  Port=2
  wires:
  Sample delay/1 -> m*/1
  Sample delay1/1 -> m/1
  Voltage Sensor/2(m) -> Sample delay1/1
  Voltage Sensor/1(m*) -> Sample delay/1
  connections:
  -/RConn1 -- Voltage Sensor/LConn2
  +/RConn1 -- Voltage Sensor/LConn1

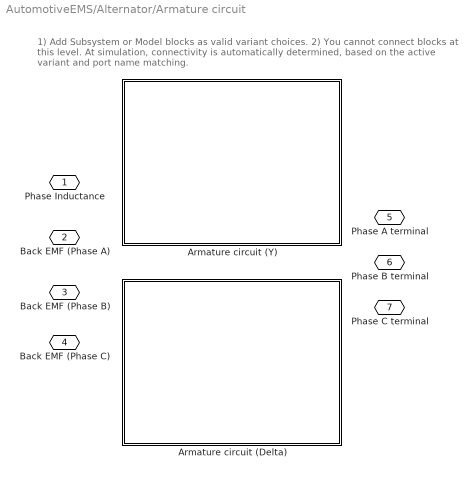
== system AutomotiveEMS/Alternator/Armature circuit ==
  note: 1) Add Subsystem or Model blocks as valid variant choices.
      | 2) You cannot connect blocks at this level. At simulation, connectivity is automatically
      | determined, based on the active variant and port name matching.
  Armature circuit (Delta) : Subsystem  VariantControl=deltaStatorConnection
  Armature circuit (Y) : Subsystem  VariantControl=yStatorConnection
  Phase Inductance : PMIOPort  Side=Left
  Back EMF (Phase A) : PMIOPort  Port=2  Side=Left
  Back EMF (Phase B) : PMIOPort  Port=3  Side=Left
  Back EMF (Phase C) : PMIOPort  Port=4  Side=Left
  Phase A terminal : PMIOPort  Port=5  Side=Right
  Phase B terminal : PMIOPort  Port=6  Side=Right
  Phase C terminal : PMIOPort  Port=7  Side=Right
